simulink model "Model_XInput"  (R2019a)
settings: Solver=FixedStepAuto  StartTime=0.0  StopTime=100  FixedStep=0.001  RelTol=1e-3
settings Model: EnablePacing=on  Creator=Mathias Voigt  LastModifiedBy=Mathias Voigt

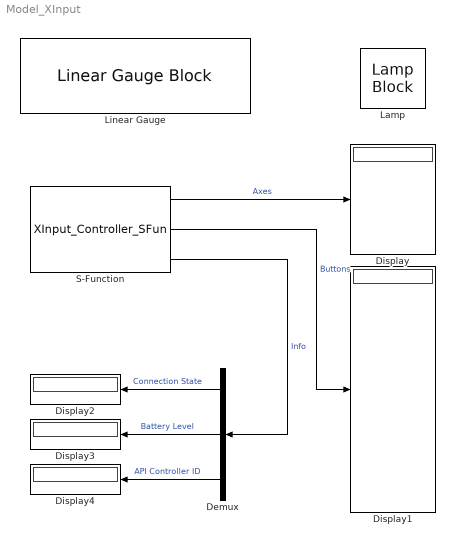
== system Model_XInput ==
  Demux : Demux  Outputs=3
  Display{,1..4} (5 alike) : Display
  Lamp : LampBlock
  Linear Gauge : LinearGaugeBlock  TickInterval=25
  S-Function : S-Function  FunctionName=XInput_Controller_SFun  Parameters=1  SFunctionDeploymentMode=off  EnableBusSupport=off
  wires:
  S-Function/2 -> Display1/1  "Buttons"
  S-Function/1 -> Display/1  "Axes"
  Demux/1 -> Display2/1  "Connection State"
  Demux/2 -> Display3/1  "Battery Level"
  Demux/3 -> Display4/1  "API Controller ID"
  S-Function/3 -> Demux/1  "Info"
